simulink model "sedemo_dist_processing_nominal"  (Simulink 7.5)
settings: Solver=VariableStepDiscrete  StartTime=0.0  StopTime=1  MaxStep=inf  RelTol=1e-3
undefined symbols (not defined in the file or in its folder): des_figposition, des_subsystemblock, des_subsysteminport, des_subsystemoutport, des_subsystemsupportblock
libraries: simeventsrouting1 x5, simeventssink1 x5, simeventsattributes2 x5, simeventsserver1 x5, simulink x3, simeventsqueue1 x3, simeventstranslate1 x1, simeventsinfo x1, simeventsgenerators1 x1
settings Model: Creator=The MathWorks Inc.
settings DataIOCC: SaveOutput=off  SaveTime=off
settings DebuggingCC: AlgebraicLoopMsg=error  SolverPrmCheckMsg=none  StrictBusMsg=Warning
settings SimEventsCC: propDiagAttribOutput=1  propDiagFcnCallOutput=1  propDiagStatOutput=0

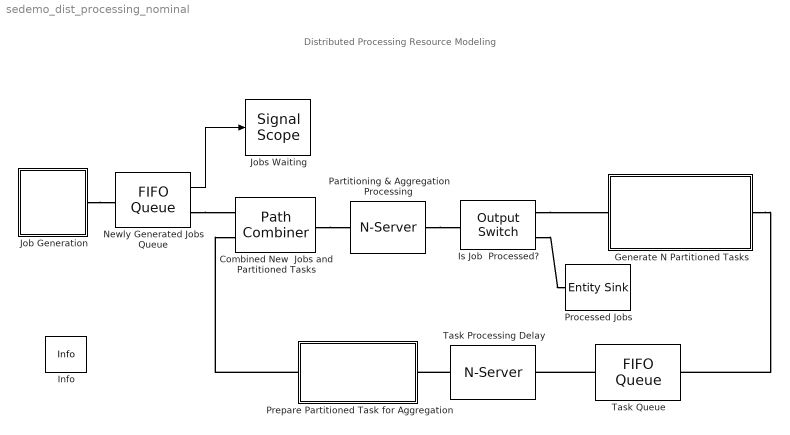
== system sedemo_dist_processing_nominal ==
  note: Distributed Processing Resource Modeling
  Combined New  Jobs and Partitioned Tasks : simeventsrouting1/Path Combiner  Priority=1  SystemSampleTime=-1  NumberInputPorts=2  InputPortPrecedence=IN1 port  InitialSeed=45675  SpecifyEventPriority=off  PriorityPathCombinerPortPrecedenceSelection=4100  StatNumberDeparted=Off  StatLastArrivalPort=Off  EvaluatedNumPorts=2
  Generate N Partitioned Tasks : Subsystem
  Info : simeventsinfo/Info  SystemSampleTime=-1
  Is Job  Processed? : simeventsrouting1/Output Switch  Priority=1  SystemSampleTime=-1  NumberOutputPorts=2  SwitchingCriterion=From attribute  InitialSeed=34567  AttributeName=Aggregation_Flag  InitialConditionsOpt=off  InitialConditions=1  EntityBufferOpt=off  SpecifyEventPriority=off  PriorityOutputSwitchSelectPort=4100  TimeoutPortOpt=off  StatNumberDeparted=Off  StatNumberTimedOut=Off  StatPendingEntity=Off  StatLastDeparturePort=Off  EvaluatedNumPorts=2
  Job Generation : Subsystem
  Jobs Waiting : simeventssink1/Signal Scope  Priority=1  SystemSampleTime=-1  PlotType=Stair  InputType=Signal  NumInputs=1  AttributeNameY=Count  XInputOptionSignal=Event time  XInputOptionEntity=Event time  AttributeNameX=Count  EnableEntityOutport=on  XMin=0  XMax=1  XLimitExceededOption=Stretch axis limits  YLimitExceededOption=Stretch axis limits  AxisGrid=on  AxisLegend=off  LineDisables=""  LineColors=[1 0 0]  LineStyles=-  LineMarkers=.  OpenScopeAtSimStart=on  Title=Jobs Waiting In Queue  YLabel=""  XLabel=Time  FigurePosition=des_figposition([35,7,30,30]);  AxisZoom=off  DataStoreOption=Limited  DataPointsLimit=10000  StatNumberArrived=Off  ShowCountPlotted=off  ShowToolbar=on
      settings: YMin=0  YMax=10
  Newly Generated Jobs Queue : simeventsqueue1/FIFO Queue  Priority=1  SystemSampleTime=-1  Capacity=inf  EnableTOPort=off  StatNumberDeparted=Off  StatNumberInBlock=On  StatPendingEntity=Off  StatAverageWait=Off  StatAverageQueueLength=Off  StatNumberTimedout=Off
  Partitioning & Aggregation Processing : simeventsserver1/N-Server  Priority=1  SystemSampleTime=-1  NumberOfServers=1  ServiceTimeFrom=Attribute  ServiceTime=1  AttributeName=Partitioning_Time  PriorityServiceCompletion=500  EnableTOPort=off  StatNumberDeparted=Off  StatNumberInBlock=Off  StatPendingEntity=Off  StatNumberPending=Off  StatAverageWait=Off  StatUtilization=Off  StatNumberTimedout=Off
      settings: AttributesFormatString=# of Servers = %<NumberOfServers>
  Prepare Partitioned Task for Aggregation : Subsystem
  Processed Jobs : simeventssink1/Entity Sink  Priority=1  SystemSampleTime=-1  AvailableForArrivals=on  StatNumberArrived=Off
  Task Processing Delay : simeventsserver1/N-Server  Priority=1  SystemSampleTime=-1  NumberOfServers=128  ServiceTimeFrom=Attribute  ServiceTime=1  AttributeName=Processing_Time  PriorityServiceCompletion=500  EnableTOPort=off  StatNumberDeparted=Off  StatNumberInBlock=Off  StatPendingEntity=Off  StatNumberPending=Off  StatAverageWait=Off  StatUtilization=Off  StatNumberTimedout=Off
      settings: AttributesFormatString=# of Servers = %<NumberOfServers>
  Task Queue : simeventsqueue1/FIFO Queue  Priority=1  SystemSampleTime=-1  Capacity=128  EnableTOPort=off  StatNumberDeparted=Off  StatNumberInBlock=Off  StatPendingEntity=Off  StatAverageWait=Off  StatAverageQueueLength=Off  StatNumberTimedout=Off
      settings: AttributesFormatString=Queue Length = %<Capacity>
  wires:
  Newly Generated Jobs Queue/1 -> Jobs Waiting/1
  connections:
  Task Queue/RConn1 -- Task Processing Delay/LConn1
  Prepare Partitioned Task for Aggregation/RConn1 -- Combined New  Jobs and Partitioned Tasks/LConn2
  Is Job  Processed?/RConn2 -- Processed Jobs/LConn1
  Generate N Partitioned Tasks/RConn1 -- Task Queue/LConn1
  Combined New  Jobs and Partitioned Tasks/RConn1 -- Partitioning & Aggregation Processing/LConn1
  Task Processing Delay/RConn1 -- Prepare Partitioned Task for Aggregation/LConn1
  Newly Generated Jobs Queue/RConn1 -- Combined New  Jobs and Partitioned Tasks/LConn1
  Partitioning & Aggregation Processing/RConn1 -- Is Job  Processed?/LConn1
  Job Generation/LConn1 -- Newly Generated Jobs Queue/LConn1
  Is Job  Processed?/RConn1 -- Generate N Partitioned Tasks/LConn1

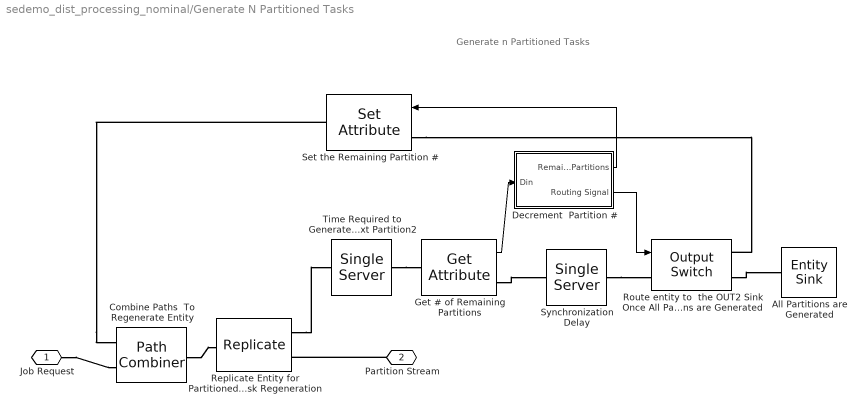
== system sedemo_dist_processing_nominal/Generate N Partitioned Tasks ==
  note: Generate n Partitioned Tasks
  All Partitions are Generated : simeventssink1/Entity Sink  Priority=1  SystemSampleTime=-1  AvailableForArrivals=on  StatNumberArrived=Off
  Combine Paths  To Regenerate Entity : simeventsrouting1/Path Combiner  Priority=1  SystemSampleTime=-1  NumberInputPorts=2  InputPortPrecedence=IN1 port  InitialSeed=45675  SpecifyEventPriority=off  PriorityPathCombinerPortPrecedenceSelection=4100  StatNumberDeparted=Off  StatLastArrivalPort=Off  EvaluatedNumPorts=2
  Decrement  Partition # : Subsystem  LoadFcn=des_subsystemblock(gcb, 'load');  InitFcn=des_subsystemblock(gcb, 'init');  StartFcn=des_subsystemblock(gcb, 'start');  StopFcn=des_subsystemblock(gcb, 'stop');
      settings: CopyFcn=des_subsystemblock(gcb, 'copy');  DeleteFcn=des_subsystemblock(gcb, 'delete');  UndoDeleteFcn=des_subsystemblock(gcb, 'undodelete');  ModelCloseFcn=des_subsystemblock(gcb, 'modelclose');  PreSaveFcn=des_subsystemblock(gcb, 'presave');  NameChangeFcn=des_subsystemblock(gcb, 'namechange');  OpenFcn=des_subsystemblock(gcb, 'open');  ParentCloseFcn=des_subsystemblock(gcb, 'parentclose');  ErrorFcn=des_subsystemerror
      mask Type: Discrete Event Subsystem
      mask Help: helpview(simeventsbhelp);
  Get # of Remaining Partitions : simeventsattributes2/Get Attribute  Priority=1  DialogController=des_ddg_create  DialogControllerArgs=DataTag12  SystemSampleTime=-1  AttributeName=Partition_Count  AttributeMissing=Error  AttributeDefaultValue=0  AttributeSendTiming=After entity departure  AttributeTreatAsVector=1  StatNumberDeparted=Off  EvaluatedDefaultAttributeValue={[]}
  Replicate Entity for Partitioned Task Regeneration : simeventsrouting1/Replicate  Priority=1  SystemSampleTime=-1  NumberOutputPorts=2  ReplicateEntityWhen=All entity output ports are not blocked  OutputPortPrecedence=OUT1 port  InitialSeed=56789  ActionUponBlocking=Discard entity  StatNumberArrived=Off  StatNumberDeparted=Off  EvaluatedNumPorts=2
  Route entity to  the OUT2 Sink Once All Partitions are Generated : simeventsrouting1/Output Switch  Priority=1  SystemSampleTime=-1  NumberOutputPorts=2  SwitchingCriterion=From signal port p  InitialSeed=34567  AttributeName=Attribute1  InitialConditionsOpt=off  InitialConditions=1  EntityBufferOpt=on  SpecifyEventPriority=off  PriorityOutputSwitchSelectPort=4100  TimeoutPortOpt=off  StatNumberDeparted=Off  StatNumberTimedOut=Off  StatPendingEntity=Off  StatLastDeparturePort=Off  EvaluatedNumPorts=2
  Set the Remaining Partition # : simeventsattributes2/Set Attribute  Priority=1  DialogController=des_ddg_create  DialogControllerArgs=DataTag16  SystemSampleTime=-1  AttributeFrom=Signal port  AttributeName=Partition_Count  AttributeTreatAsVector=1  AttributeValue=0  AttributeCreate=on  StatNumberDeparted=Off  EvaluatedAttributeValue={[]}
  Synchronization Delay : simeventsserver1/Single Server  Priority=1  SystemSampleTime=-1  ServiceTimeFrom=Dialog  ServiceTime=0  AttributeName=xyz  PriorityServiceCompletion=500  PermitPreemption=off  SortingAttributeName=PriorityAttributeName  SortingDirection=Ascending  WriteToAttribute=off  ResidualAttributeName=ResidualServiceTime  CreateAttribute=on  EnableTOPort=off  StatNumberDeparted=Off  StatNumberInBlock=Off  StatNumberPreempted=Off  StatPendingEntity=Off  StatAverageWait=Off  StatUtilization=Off  StatNumberTimedout=Off
  Time Required to Generate Next Partition2 : simeventsserver1/Single Server  Priority=1  SystemSampleTime=-1  ServiceTimeFrom=Attribute  ServiceTime=0  AttributeName=Interpartition_Time  PriorityServiceCompletion=500  PermitPreemption=off  SortingAttributeName=PriorityAttributeName  SortingDirection=Ascending  WriteToAttribute=off  ResidualAttributeName=ResidualServiceTime  CreateAttribute=on  EnableTOPort=off  StatNumberDeparted=Off  StatNumberInBlock=Off  StatNumberPreempted=Off  StatPendingEntity=Off  StatAverageWait=Off  StatUtilization=Off  StatNumberTimedout=Off
  Job Request : PMIOPort  Port=1  Side=Left
  Partition Stream : PMIOPort  Port=2  Side=Right
  wires:
  Get # of Remaining Partitions/1 -> Decrement  Partition #/1(Din)
  Decrement  Partition #/2(Routing Signal) -> Route entity to  the OUT2 Sink Once All Partitions are Generated/1
  Decrement  Partition #/1(Remaining Partitions) -> Set the Remaining Partition #/1
  connections:
  Route entity to  the OUT2 Sink Once All Partitions are Generated/RConn2 -- All Partitions are Generated/LConn1
  Combine Paths  To Regenerate Entity/RConn1 -- Replicate Entity for Partitioned Task Regeneration/LConn1
  Partition Stream/RConn1 -- Replicate Entity for Partitioned Task Regeneration/RConn2
  Time Required to Generate Next Partition2/RConn1 -- Get # of Remaining Partitions/LConn1
  Replicate Entity for Partitioned Task Regeneration/RConn1 -- Time Required to Generate Next Partition2/LConn1
  Job Request/RConn1 -- Combine Paths  To Regenerate Entity/LConn2
  Set the Remaining Partition #/RConn1 -- Combine Paths  To Regenerate Entity/LConn1
  Set the Remaining Partition #/LConn1 -- Route entity to  the OUT2 Sink Once All Partitions are Generated/RConn1
  Get # of Remaining Partitions/RConn1 -- Synchronization Delay/LConn1
  Synchronization Delay/RConn1 -- Route entity to  the OUT2 Sink Once All Partitions are Generated/LConn1

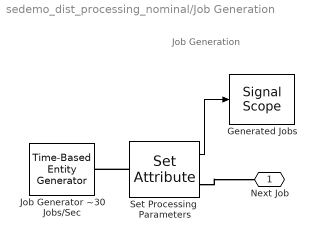
== system sedemo_dist_processing_nominal/Job Generation ==
  note: Job Generation
  Generated Jobs : simeventssink1/Signal Scope  Priority=1  SystemSampleTime=-1  PlotType=Stair  InputType=Signal  NumInputs=1  AttributeNameY=Count  XInputOptionSignal=Event time  XInputOptionEntity=Event time  AttributeNameX=Count  EnableEntityOutport=on  XMin=0  XMax=1  XLimitExceededOption=Stretch axis limits  YLimitExceededOption=Stretch axis limits  AxisGrid=on  AxisLegend=off  LineDisables=""  LineColors=b  LineStyles=-  LineMarkers=.  OpenScopeAtSimStart=on  Title=Generated Jobs  YLabel=""  XLabel=Time  FigurePosition=des_figposition([65,7,30,30]);  AxisZoom=off  DataStoreOption=Limited  DataPointsLimit=10000  StatNumberArrived=Off  ShowCountPlotted=off  ShowToolbar=on
      settings: YMin=0  YMax=10
  Job Generator ~30 Jobs/Sec : simeventsgenerators1/Entity Generators/Time-Based Entity Generator  Priority=1  DialogController=des_ddg_create  DialogControllerArgs=DataTag22  SystemSampleTime=-1  GenerateEntitiesUpon=Intergeneration time from dialog  Distribution=Constant  Minimum=0  Maximum=1  Mean=1  InitialSeed=12345  Period=0.0333  PriorityEntityGeneration=300  GenerateEntityAtSimulationStart=on  ResponseWhenBlocked=Error  ResponseWhenUnblocked=Immediate restart  EntityType=Standard  StatNumberDeparted=Off  StatPendingEntity=Off  StatAverageIntergenerationTime=Off
  Set Processing  Parameters : simeventsattributes2/Set Attribute  Priority=1  DialogController=des_ddg_create  DialogControllerArgs=DataTag24  SystemSampleTime=-1  AttributeFrom=Dialog|Dialog|Dialog|Dialog|Dialog|Dialog  AttributeName=Partition_Count|Partitioning_Time|Processing_Time|Aggregation_Flag|Interpartition_Time|Aggregation_Time  AttributeTreatAsVector=1|1|1|1|1|1  AttributeValue=256|0.0001|0.05|1| .0001|0.00005  AttributeCreate=on  StatNumberDeparted=On  EvaluatedAttributeValue={256;0.0001;0.05;1; .0001;0.00005}
  Next Job : PMIOPort  Port=1  Side=Left
  wires:
  Set Processing  Parameters/1 -> Generated Jobs/1
  connections:
  Set Processing  Parameters/LConn1 -- Job Generator ~30 Jobs/Sec/RConn1
  Set Processing  Parameters/RConn1 -- Next Job/RConn1

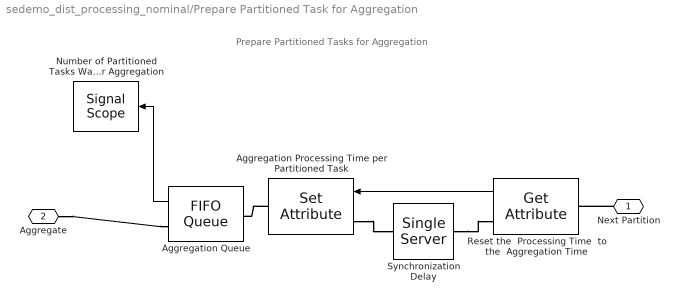
== system sedemo_dist_processing_nominal/Prepare Partitioned Task for Aggregation ==
  note: Prepare Partitioned Tasks for Aggregation
  Aggregation Processing Time per Partitioned Task : simeventsattributes2/Set Attribute  Priority=1  DialogController=des_ddg_create  DialogControllerArgs=DataTag29  SystemSampleTime=-1  AttributeFrom=Signal port|Dialog  AttributeName=Partitioning_Time|Aggregation_Flag  AttributeTreatAsVector=1|1  AttributeValue=0|2  AttributeCreate=on  StatNumberDeparted=Off  EvaluatedAttributeValue={[];2}
  Aggregation Queue : simeventsqueue1/FIFO Queue  Priority=1  SystemSampleTime=-1  Capacity=inf  EnableTOPort=off  StatNumberDeparted=Off  StatNumberInBlock=On  StatPendingEntity=Off  StatAverageWait=Off  StatAverageQueueLength=Off  StatNumberTimedout=Off
  Number of Partitioned Tasks Waiting for Aggregation : simeventssink1/Signal Scope  Priority=1  SystemSampleTime=-1  PlotType=Stair  InputType=Signal  NumInputs=1  AttributeNameY=Count  XInputOptionSignal=Event time  XInputOptionEntity=Event time  AttributeNameX=Count  EnableEntityOutport=on  XMin=0  XMax=1  XLimitExceededOption=Stretch axis limits  YLimitExceededOption=Stretch axis limits  AxisGrid=on  AxisLegend=off  LineDisables=""  LineColors=[1 0 1]  LineStyles=-  LineMarkers=None  OpenScopeAtSimStart=on  Title=Partitions Waiting For Aggregation  YLabel=""  XLabel=Time  FigurePosition=des_figposition([5,7,30,30]);  AxisZoom=off  DataStoreOption=Unlimited  DataPointsLimit=10000  StatNumberArrived=Off  ShowCountPlotted=off  ShowToolbar=on
      settings: YMin=0  YMax=10
  Reset the  Processing Time  to the  Aggregation Time : simeventsattributes2/Get Attribute  Priority=1  DialogController=des_ddg_create  DialogControllerArgs=DataTag33  SystemSampleTime=-1  AttributeName=Aggregation_Time  AttributeMissing=Error  AttributeDefaultValue=0  AttributeSendTiming=After entity departure  AttributeTreatAsVector=1  StatNumberDeparted=Off  EvaluatedDefaultAttributeValue={[]}
  Synchronization Delay : simeventsserver1/Single Server  Priority=1  SystemSampleTime=-1  ServiceTimeFrom=Dialog  ServiceTime=0  AttributeName=xyz  PriorityServiceCompletion=500  PermitPreemption=off  SortingAttributeName=PriorityAttributeName  SortingDirection=Ascending  WriteToAttribute=off  ResidualAttributeName=ResidualServiceTime  CreateAttribute=on  EnableTOPort=off  StatNumberDeparted=Off  StatNumberInBlock=Off  StatNumberPreempted=Off  StatPendingEntity=Off  StatAverageWait=Off  StatUtilization=Off  StatNumberTimedout=Off
  Next Partition : PMIOPort  Port=1  Side=Left
  Aggregate : PMIOPort  Port=2  Side=Right
  wires:
  Aggregation Queue/1 -> Number of Partitioned Tasks Waiting for Aggregation/1
  Reset the  Processing Time  to the  Aggregation Time/1 -> Aggregation Processing Time per Partitioned Task/1
  connections:
  Aggregation Processing Time per Partitioned Task/RConn1 -- Aggregation Queue/LConn1
  Next Partition/RConn1 -- Reset the  Processing Time  to the  Aggregation Time/LConn1
  Aggregate/RConn1 -- Aggregation Queue/RConn1
  Aggregation Processing Time per Partitioned Task/LConn1 -- Synchronization Delay/RConn1
  Synchronization Delay/LConn1 -- Reset the  Processing Time  to the  Aggregation Time/RConn1

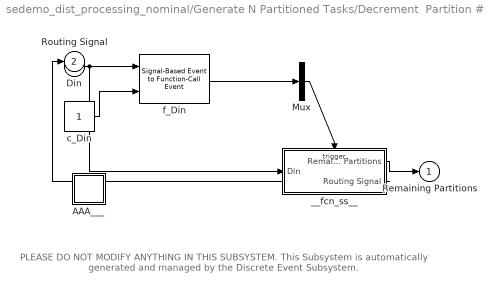
== system sedemo_dist_processing_nominal/Generate N Partitioned Tasks/Decrement  Partition # ==
  note: PLEASE DO NOT MODIFY ANYTHING IN THIS SUBSYSTEM.
      | This Subsystem is automatically generated and
      | managed by the Discrete Event Subsystem.
  Din : Inport  DataType=double  OutDataType=sfix(16)  OutScaling=2^0  OutDataTypeStr=double
  AAA___ : Subsystem  LoadFcn=des_subsystemsupportblock(gcb, 'load');  InitFcn=des_subsystemsupportblock(gcb, 'init');  StartFcn=des_subsystemsupportblock(gcb, 'start');  StopFcn=des_subsystemsupportblock(gcb, 'stop');
      settings: CopyFcn=des_subsystemsupportblock(gcb, 'copy');  DeleteFcn=des_subsystemsupportblock(gcb, 'delete');  UndoDeleteFcn=des_subsystemsupportblock(gcb, 'undodelete');  ModelCloseFcn=des_subsystemsupportblock(gcb, 'modelclose');  PreSaveFcn=des_subsystemsupportblock(gcb, 'presave');  NameChangeFcn=des_subsystemsupportblock(gcb, 'namechange');  OpenFcn=des_subsystemsupportblock(gcb, 'open');  ParentCloseFcn=des_subsystemsupportblock(gcb, 'parentclose');
  Mux : Mux  Inputs=1
  __fcn_ss__ : Subsystem  TreatAsAtomicUnit=on
      settings: PropExecContextOutsideSubsystem=on
  c_Din : Constant  OutDataType=sfix(16)  OutScaling=2^0
  f_Din : simeventstranslate1/Signal-Based Event to Function-Call Event  Priority=1  SystemSampleTime=-1  GenerateFunctionCallUpon=Change in signal from port vc  SignalEdgeOption=Either  EnableE1Port=on  EnableF2Port=off  EnableE2Port=off  SpecifyEventPriority=off  PriorityFunctionCall=20  FunctionCallDelayFrom=Dialog  DelayFunctionCall=0  StatNumberF1Calls=Off  StatNumberF2Calls=Off  MaskBlockType=DESS_EVENT_PORT
  Remaining Partitions : Outport  OutDataType=sfix(16)  OutScaling=2^0
  Routing Signal : Outport  Port=2  OutDataType=sfix(16)  OutScaling=2^0
  wires:
  __fcn_ss__/1(Remaining Partitions) -> Remaining Partitions/1
  f_Din/1 -> Mux/1
  c_Din/1 -> f_Din/2
  Mux/1 -> __fcn_ss__/Trigger
  __fcn_ss__/2(Routing Signal) -> Routing Signal/1
  Din/1 -> f_Din/1, __fcn_ss__/1(Din)

== system sedemo_dist_processing_nominal/Generate N Partitioned Tasks/Decrement  Partition #/AAA___ ==

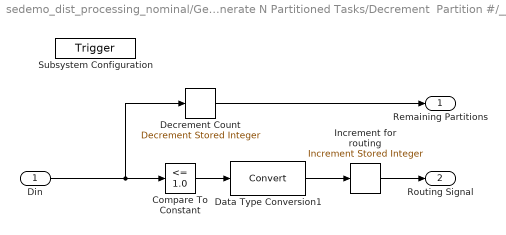
== system sedemo_dist_processing_nominal/Generate N Partitioned Tasks/Decrement  Partition #/__fcn_ss__ ==
  Din : Inport  LoadFcn=des_subsysteminport(gcb, 'load');  InitFcn=des_subsysteminport(gcb, 'init');  StartFcn=des_subsysteminport(gcb, 'start');  StopFcn=des_subsysteminport(gcb, 'stop');  OutDataType=sfix(16)  OutScaling=2^0  mask(Discrete Event Inport){PermitSubsystemEvents=on, TypeOfEvent=Change in signal, SignalEdgeOption=Either, SpecifyEventPriority=off, PrioritySubsystemEvent=20}
      mask prompts: PermitSubsystemEvents "Execute subsystem upon signal-based events"; TypeOfEvent "Type of signal-based event:"; SignalEdgeOption "Type of change in signal value:"; SpecifyEventPriority "Resolve simultaneous signal updates according to event priority"; PrioritySubsystemEvent "Event priority:"
      mask help: Input port for a Discrete Event Subsystem block. This block can conditionally execute the subsystem upon signal-based events that meet specified criteria.
      mask init:
      | des_subsystemmask(gcb, 'init','apply')
      settings: CopyFcn=des_subsysteminport(gcb, 'copy');  DeleteFcn=des_subsysteminport(gcb, 'delete');  UndoDeleteFcn=des_subsysteminport(gcb, 'undodelete');  ModelCloseFcn=des_subsysteminport(gcb, 'modelclose');  PreSaveFcn=des_subsysteminport(gcb, 'presave');  NameChangeFcn=des_subsysteminport(gcb, 'namechange');  ParentCloseFcn=des_subsysteminport(gcb, 'parentclose');
      mask Help: helpview(simeventsbhelp);
      mask StyleString: checkbox,popup(Change in signal|Trigger|Sample time hit),popup(Rising|Falling|Either),checkbox,edit
      mask CallbackString: des_subsystemmask(gcb, 'cbPermitSubsystemEvents', 'noapply');|des_subsystemmask(gcb,'cbTypeOfEvent','noapply');||des_subsystemmask(gcb, 'cbSpecifyEventPriority', 'noapply');|
  Subsystem Configuration : TriggerPort  TriggerType=function-call
      settings: CopyFcn=des_subsystemconfigblock(gcb, 'copy');  DeleteFcn=des_subsystemconfigblock(gcb, 'delete');  UndoDeleteFcn=des_subsystemconfigblock(gcb, 'undodelete');
      mask Type: Subsystem Configuration
      mask Description: Configuration for a Discrete Event Subsystem block. Every discrete event subsystem window must contain exactly one copy of this configuration block. Do not delete this block.
      mask Help: helpview(simeventsbhelp);
      mask Display: disp('Do Not Delete');
  Compare To Constant : simulink/Logic and Bit Operations/Compare To Constant  SystemSampleTime=-1  relop=<=  const=1.0  LogicOutDataTypeMode=uint8  ZeroCross=off
  Data Type Conversion1 : DataTypeConversion  OutDataType=sfix(16)  OutScaling=2^0
  Decrement Count : simulink/Additional Math & Discrete/Additional Math: Increment - Decrement/Decrement Stored Integer  SystemSampleTime=-1
  Increment for routing : simulink/Additional Math & Discrete/Additional Math: Increment - Decrement/Increment Stored Integer  SystemSampleTime=-1
  Remaining Partitions : Outport  LoadFcn=des_subsystemoutport(gcb, 'load');  InitFcn=des_subsystemoutport(gcb, 'init');  StartFcn=des_subsystemoutport(gcb, 'start');  StopFcn=des_subsystemoutport(gcb, 'stop');  OutDataType=sfix(16)  OutScaling=2^0  mask(Discrete Event Outport){InitOutput=[]}
      mask prompts: InitOutput "Initial output:"
      mask help: Provide an output port for a Discrete Event Subsystem block.
      settings: CopyFcn=des_subsystemoutport(gcb, 'copy');  DeleteFcn=des_subsystemoutport(gcb, 'delete');  UndoDeleteFcn=des_subsystemoutport(gcb, 'undodelete');  ModelCloseFcn=des_subsystemoutport(gcb, 'modelclose');  PreSaveFcn=des_subsystemoutport(gcb, 'presave');  NameChangeFcn=des_subsystemoutport(gcb, 'namechange');  ParentCloseFcn=des_subsystemoutport(gcb, 'parentclose');
      mask Help: helpview(simeventsbhelp);
      mask CallbackString: set_param(gcb,'InitialOutput',get_param(gcb,'InitOutput'));
  Routing Signal : Outport  LoadFcn=des_subsystemoutport(gcb, 'load');  InitFcn=des_subsystemoutport(gcb, 'init');  StartFcn=des_subsystemoutport(gcb, 'start');  StopFcn=des_subsystemoutport(gcb, 'stop');  Port=2  OutDataType=sfix(16)  OutScaling=2^0  mask(Discrete Event Outport){InitOutput=[]}
      mask prompts: InitOutput "Initial output:"
      mask help: Provide an output port for a Discrete Event Subsystem block.
      settings: CopyFcn=des_subsystemoutport(gcb, 'copy');  DeleteFcn=des_subsystemoutport(gcb, 'delete');  UndoDeleteFcn=des_subsystemoutport(gcb, 'undodelete');  ModelCloseFcn=des_subsystemoutport(gcb, 'modelclose');  PreSaveFcn=des_subsystemoutport(gcb, 'presave');  NameChangeFcn=des_subsystemoutport(gcb, 'namechange');  ParentCloseFcn=des_subsystemoutport(gcb, 'parentclose');
      mask Help: helpview(simeventsbhelp);
      mask CallbackString: set_param(gcb,'InitialOutput',get_param(gcb,'InitOutput'));
  wires:
  Compare To Constant/1 -> Data Type Conversion1/1
  Data Type Conversion1/1 -> Increment for routing/1
  Increment for routing/1 -> Routing Signal/1
  Decrement Count/1 -> Remaining Partitions/1
  Din/1 -> Compare To Constant/1, Decrement Count/1
